simulink model "rcm112_app"  (R2024a)
settings: Solver=FixedStepDiscrete  StartTime=0.0  StopTime=10.0  FixedStep=0.005  RelTol=1e-3  EnableMultiTasking=on
PreLoadFcn:
  | try, model_open; catch, disp('Error occurred while executing model pre-load callback: model_open.m'); disp('Please assure that the MATLAB working directory is set to the model directory before opening.'); end
InitFcn:
  | try, model_open; catch, end
undefined symbols (not defined in the file or in its folder): dataName, enumName, enumValue, raptor_get_safe_string, raptor_xcp_function, RCM
libraries: Raptor_lib x57, simulink x14, simulink_extras x4
(part 2 of 2)

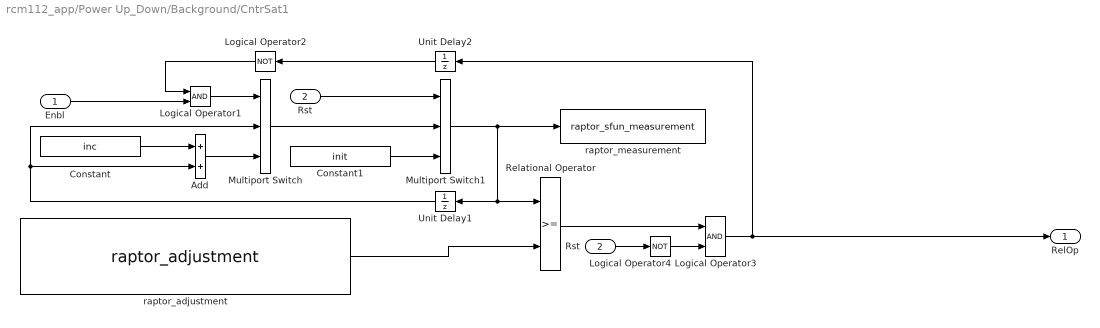
== system rcm112_app/Power Up_Down/Background/CntrSat1 ==
  Enbl : Inport
  Rst : Inport  Port=2
  Add : Sum  InputSameDT=on  OutDataTypeStr=Inherit: Same as first input
  Constant : Constant  Value=inc  OutDataTypeStr=uint32
  Constant1 : Constant  Value=init  OutDataTypeStr=uint32
  Logical Operator1 : Logic  OutDataTypeStr=boolean
  Logical Operator2 : Logic  Operator=NOT  Inputs=1  OutDataTypeStr=boolean
  Logical Operator3 : Logic  OutDataTypeStr=boolean
  Logical Operator4 : Logic  Operator=NOT  Inputs=1  OutDataTypeStr=boolean
  Multiport Switch : MultiPortSwitch  DataPortOrder=Zero-based contiguous  Inputs=2  zeroidx=on  SaturateOnIntegerOverflow=off
  Multiport Switch1 : MultiPortSwitch  DataPortOrder=Zero-based contiguous  Inputs=2  zeroidx=on  SaturateOnIntegerOverflow=off
  Relational Operator : RelationalOperator  OutDataTypeStr=boolean  InputSameDT=off
  "Rst " : InportShadow  Port=2
  Unit Delay1 : UnitDelay  InitialCondition=init  SampleTime=-1  HasFrameUpgradeWarning=on
  Unit Delay2 : UnitDelay  InitialCondition=boolean(0)  SampleTime=-1  HasFrameUpgradeWarning=on
  raptor_adjustment : Raptor_lib/Data Storage/raptor_adjustment  paramName=th_nam  nameSource=Parameter  initValue=timeout / th_gain  dataType=uint32  storage=Calibration  calDispType=Number  calEnum={'Disabled', 'Enabled'}  calGain=th_gain  calOffset=0  calMax=inf  calMin=-inf  calFormat='0.3'  calUnit=th_units  calHelp=th_help  calAccess=4  calFunction=th_group  calDispHeaders=off  calColHeaders={'Col1' 'Col2' 'Col3'}  calRowHeaders={'Row1' 'Row2' 'Row3'}
      settings: SourceProductName=Raptor
  raptor_measurement : S-Function  FunctionName=raptor_sfun_measurement  Parameters=char({dataName,''}), uint8(calDispType), char(enumName), int32(enumValue), double(calGain), double(calOffset), double(calMax), double(calMin), char(calUnit), char(calHelp), char(calFormat), char(calFunction), char(calAccess)  SFunctionDeploymentMode=off  EnableBusSupport=off  mask(Measurement){paramName=[th_nam(1:end-3) 'Tmr'], nameSource=Parameter, calDispType=Number, calEnum={'False', 'True'}, calGain=th_gain, calOffset=0.0, calMax=inf, calMin=-inf, calFormat='0.3', calUnit=th_units, calHelp=['time that gets compared to ' th_nam], calAccess=4, calFunction=th_group, calVisible=on}
      mask prompts: paramName "Name"; nameSource "Name Source"; calDispType "Display as"; calEnum "Enumeration Definition"; calGain "Gain"; calOffset "Offset"; calMax "Max"; calMin "Min"; calFormat "Display Decimal Places"; calUnit "Unit Text"; calHelp "Help Text"; calAccess "Access Level"; calFunction "Function"; calVisible "Visible in Cal"
      mask help: This block is used to display a value in the calibration tool.
      mask init:
      | raptor_sfun_measurement_maskInit;
      settings: MoveFcn=raptor_icon_redraw(gcb);
      mask Help: eval('raptor_help(''raptor_measurement'');')
      mask TypeOptions nameSource: Parameter | Input Wire
      mask Callback nameSource: raptor_sfun_measurement_dlgCb(gcb, 'nameSource');
      mask TypeOptions calDispType: Number | Enumeration | String
      mask Callback calDispType: raptor_sfun_measurement_dlgCb(gcb, 'calDispType');
      mask TypeOptions calAccess: 4 | 3 | 2 | 1
      mask Display: raptor_sfun_measurement_icon;
  RelOp : Outport  VectorParamsAs1DForOutWhenUnconnected=off
  wires:
  "Rst "/1 -> Logical Operator4/1
  Logical Operator4/1 -> Logical Operator3/2
  Relational Operator/1 -> Logical Operator3/1
  Multiport Switch1/1 -> Relational Operator/1, Unit Delay1/1, raptor_measurement/1
  Logical Operator2/1 -> Logical Operator1/1
  Constant1/1 -> Multiport Switch1/3
  Multiport Switch/1 -> Multiport Switch1/2
  Constant/1 -> Add/1
  Unit Delay1/1 -> Multiport Switch/2, Add/2
  Add/1 -> Multiport Switch/3
  Logical Operator1/1 -> Multiport Switch/1
  Enbl/1 -> Logical Operator1/2
  raptor_adjustment/1 -> Relational Operator/2
  Logical Operator3/1 -> RelOp/1, Unit Delay2/1
  Rst/1 -> Multiport Switch1/1
  Unit Delay2/1 -> Logical Operator2/1

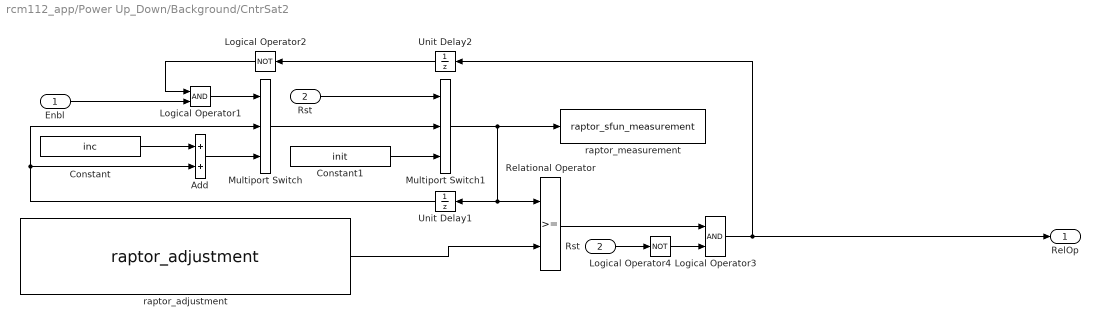
== system rcm112_app/Power Up_Down/Background/CntrSat2 ==
  Enbl : Inport
  Rst : Inport  Port=2
  Add : Sum  InputSameDT=on  OutDataTypeStr=Inherit: Same as first input
  Constant : Constant  Value=inc  OutDataTypeStr=uint32
  Constant1 : Constant  Value=init  OutDataTypeStr=uint32
  Logical Operator1 : Logic  OutDataTypeStr=boolean
  Logical Operator2 : Logic  Operator=NOT  Inputs=1  OutDataTypeStr=boolean
  Logical Operator3 : Logic  OutDataTypeStr=boolean
  Logical Operator4 : Logic  Operator=NOT  Inputs=1  OutDataTypeStr=boolean
  Multiport Switch : MultiPortSwitch  DataPortOrder=Zero-based contiguous  Inputs=2  zeroidx=on  SaturateOnIntegerOverflow=off
  Multiport Switch1 : MultiPortSwitch  DataPortOrder=Zero-based contiguous  Inputs=2  zeroidx=on  SaturateOnIntegerOverflow=off
  Relational Operator : RelationalOperator  OutDataTypeStr=boolean  InputSameDT=off
  "Rst " : InportShadow  Port=2
  Unit Delay1 : UnitDelay  InitialCondition=init  SampleTime=-1  HasFrameUpgradeWarning=on
  Unit Delay2 : UnitDelay  InitialCondition=boolean(0)  SampleTime=-1  HasFrameUpgradeWarning=on
  raptor_adjustment : Raptor_lib/Data Storage/raptor_adjustment  paramName=th_nam  nameSource=Parameter  initValue=timeout / th_gain  dataType=uint32  storage=Calibration  calDispType=Number  calEnum={'Disabled', 'Enabled'}  calGain=th_gain  calOffset=0  calMax=inf  calMin=-inf  calFormat='0.3'  calUnit=th_units  calHelp=th_help  calAccess=4  calFunction=th_group  calDispHeaders=off  calColHeaders={'Col1' 'Col2' 'Col3'}  calRowHeaders={'Row1' 'Row2' 'Row3'}
      settings: SourceProductName=Raptor
  raptor_measurement : S-Function  FunctionName=raptor_sfun_measurement  Parameters=char({dataName,''}), uint8(calDispType), char(enumName), int32(enumValue), double(calGain), double(calOffset), double(calMax), double(calMin), char(calUnit), char(calHelp), char(calFormat), char(calFunction), char(calAccess)  SFunctionDeploymentMode=off  EnableBusSupport=off  mask(Measurement){paramName=[th_nam(1:end-3) 'Tmr'], nameSource=Parameter, calDispType=Number, calEnum={'False', 'True'}, calGain=th_gain, calOffset=0.0, calMax=inf, calMin=-inf, calFormat='0.3', calUnit=th_units, calHelp=['time that gets compared to ' th_nam], calAccess=4, calFunction=th_group, calVisible=on}
      mask prompts: paramName "Name"; nameSource "Name Source"; calDispType "Display as"; calEnum "Enumeration Definition"; calGain "Gain"; calOffset "Offset"; calMax "Max"; calMin "Min"; calFormat "Display Decimal Places"; calUnit "Unit Text"; calHelp "Help Text"; calAccess "Access Level"; calFunction "Function"; calVisible "Visible in Cal"
      mask help: This block is used to display a value in the calibration tool.
      mask init:
      | raptor_sfun_measurement_maskInit;
      settings: MoveFcn=raptor_icon_redraw(gcb);
      mask Help: eval('raptor_help(''raptor_measurement'');')
      mask TypeOptions nameSource: Parameter | Input Wire
      mask Callback nameSource: raptor_sfun_measurement_dlgCb(gcb, 'nameSource');
      mask TypeOptions calDispType: Number | Enumeration | String
      mask Callback calDispType: raptor_sfun_measurement_dlgCb(gcb, 'calDispType');
      mask TypeOptions calAccess: 4 | 3 | 2 | 1
      mask Display: raptor_sfun_measurement_icon;
  RelOp : Outport  VectorParamsAs1DForOutWhenUnconnected=off
  wires:
  "Rst "/1 -> Logical Operator4/1
  Logical Operator4/1 -> Logical Operator3/2
  Relational Operator/1 -> Logical Operator3/1
  Multiport Switch1/1 -> Relational Operator/1, Unit Delay1/1, raptor_measurement/1
  Logical Operator2/1 -> Logical Operator1/1
  Constant1/1 -> Multiport Switch1/3
  Multiport Switch/1 -> Multiport Switch1/2
  Constant/1 -> Add/1
  Unit Delay1/1 -> Multiport Switch/2, Add/2
  Add/1 -> Multiport Switch/3
  Logical Operator1/1 -> Multiport Switch/1
  Enbl/1 -> Logical Operator1/2
  raptor_adjustment/1 -> Relational Operator/2
  Logical Operator3/1 -> RelOp/1, Unit Delay2/1
  Rst/1 -> Multiport Switch1/1
  Unit Delay2/1 -> Logical Operator2/1

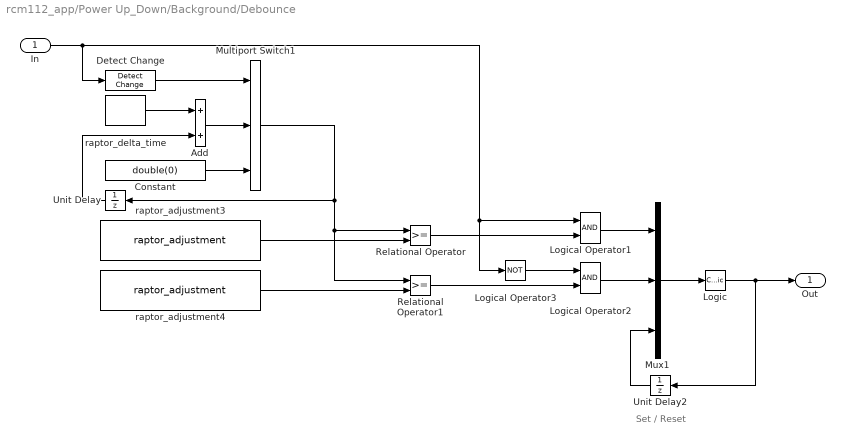
== system rcm112_app/Power Up_Down/Background/Debounce ==
  note: Set / Reset
  In : Inport
  Add : Sum
  Constant : Constant  Value=double(0)
  Detect Change : simulink/Logic and Bit Operations/Detect Change  vinit=0  OutDataTypeStr=boolean
  Logic : CombinatorialLogic  TruthTable=[0;1;0;0;1;1;0;0]
  Logical Operator1 : Logic  AllPortsSameDT=off  OutDataTypeStr=boolean
  Logical Operator2 : Logic  AllPortsSameDT=off  OutDataTypeStr=boolean
  Logical Operator3 : Logic  Operator=NOT  Inputs=1  AllPortsSameDT=off  OutDataTypeStr=boolean
  Multiport Switch1 : MultiPortSwitch  DataPortOrder=Zero-based contiguous  Inputs=2  zeroidx=on  SaturateOnIntegerOverflow=off  InputSameDT=off
  Mux1 : Mux  Inputs=3
  Relational Operator : RelationalOperator  OutDataTypeStr=boolean  InputSameDT=off
  Relational Operator1 : RelationalOperator  OutDataTypeStr=boolean  InputSameDT=off
  Unit Delay : UnitDelay  SampleTime=-1  HasFrameUpgradeWarning=on
  Unit Delay2 : UnitDelay  InitialCondition=1  SampleTime=-1  HasFrameUpgradeWarning=on
  raptor_adjustment3 : Raptor_lib/Data Storage/raptor_adjustment  paramName='KeySwHiTimeThr'  nameSource=Parameter  initValue=0.2  dataType=double  storage=Calibration  calDispType=Number  calEnum={'Active Low', 'Active High'}  calGain=1  calOffset=0  calMax=inf  calMin=-inf  calFormat='-1'  calUnit='sec'  calHelp='State high time threshold'  calAccess=1  calFunction=group  calDispHeaders=off  calColHeaders={'Col1' 'Col2' 'Col3'}  calRowHeaders={'Row1' 'Row2' 'Row3'}
      settings: SourceProductName=Raptor
  raptor_adjustment4 : Raptor_lib/Data Storage/raptor_adjustment  paramName='KeySwLoTimeThr'  nameSource=Parameter  initValue=0.2  dataType=double  storage=Calibration  calDispType=Number  calEnum={'Active Low', 'Active High'}  calGain=1  calOffset=0  calMax=inf  calMin=-inf  calFormat='-1'  calUnit='sec'  calHelp='State low time threshold'  calAccess=1  calFunction=group  calDispHeaders=off  calColHeaders={'Col1' 'Col2' 'Col3'}  calRowHeaders={'Row1' 'Row2' 'Row3'}
      settings: SourceProductName=Raptor
  raptor_delta_time : Raptor_lib/Triggers/raptor_delta_time  unit=seconds
      settings: SourceProductName=Raptor
  Out : Outport  VectorParamsAs1DForOutWhenUnconnected=off
  wires:
  Detect Change/1 -> Multiport Switch1/1
  Logical Operator3/1 -> Logical Operator2/1
  Relational Operator/1 -> Logical Operator1/2
  Logical Operator2/1 -> Mux1/2
  Logical Operator1/1 -> Mux1/1
  Mux1/1 -> Logic/1
  Unit Delay2/1 -> Mux1/3
  In/1 -> Detect Change/1, Logical Operator1/1, Logical Operator3/1
  Multiport Switch1/1 -> Unit Delay/1, Relational Operator/1, Relational Operator1/1
  Add/1 -> Multiport Switch1/2
  Constant/1 -> Multiport Switch1/3
  Relational Operator1/1 -> Logical Operator2/2
  Logic/1 -> Unit Delay2/1, Out/1
  Unit Delay/1 -> Add/2
  raptor_delta_time/1 -> Add/1
  raptor_adjustment4/1 -> Relational Operator1/2
  raptor_adjustment3/1 -> Relational Operator/2

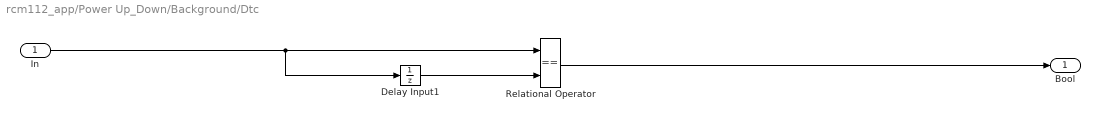
== system rcm112_app/Power Up_Down/Background/Dtc ==
  In : Inport
  Delay Input1 : UnitDelay  Description=Store in Global RAM  DisableCoverage=on  InitialCondition=init  SampleTime=-1  HasFrameUpgradeWarning=on
  Relational Operator : RelationalOperator  Operator===  OutDataTypeStr=boolean
  Bool : Outport  InitialOutput=0  VectorParamsAs1DForOutWhenUnconnected=off
  wires:
  In/1 -> Delay Input1/1, Relational Operator/1
  Delay Input1/1 -> Relational Operator/2
  Relational Operator/1 -> Bool/1

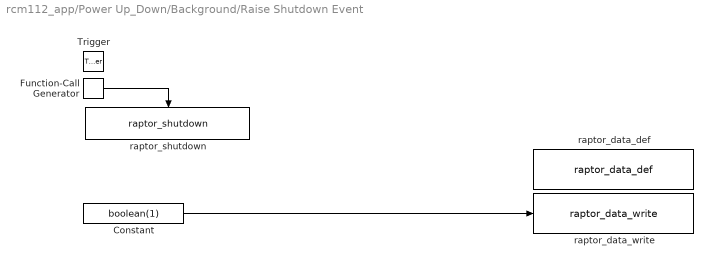
== system rcm112_app/Power Up_Down/Background/Raise Shutdown Event ==
  Trigger : TriggerPort  TriggerType=falling  VariantControl=Variant
  Constant : Constant  Value=boolean(1)
  Function-Call Generator : simulink/Ports & Subsystems/Function-Call Generator  sample_time=-1  numberOfIterations=1  DisallowWideOutput=off
  raptor_data_def : Raptor_lib/Data Storage/raptor_data_def  dataName='FgndTasksStopped'  initValue=0  dataType=boolean  storage=Volatile (RAM)  calVisible=on  calType=Measurement  calDispType=Number  calEnum={'False', 'True'}  calGain=1.0  calOffset=0  calMin=-Inf  calMax=Inf  calFormat='-1'  calUnit='Bool'  calHelp='Boolean indicating foreground tasks stopped'  calAccess=1  calFunction=group  calDispHeaders=off  calColHeaders={'Col1' 'Col2' 'Col3'}  calRowHeaders={'Row1' 'Row2' 'Row3'}
      settings: SourceProductName=Raptor
  raptor_data_write : Raptor_lib/Data Storage/raptor_data_write  dataName='FgndTasksStopped'  dataShape=Scalar  idxSource=Input Port  idxRow=1  idxCol=1
      settings: SourceProductName=Raptor
  raptor_shutdown : Raptor_lib/Triggers/raptor_shutdown  null=0
      settings: SourceProductName=Raptor
  wires:
  Constant/1 -> raptor_data_write/1
  Function-Call Generator/1 -> raptor_shutdown/Trigger

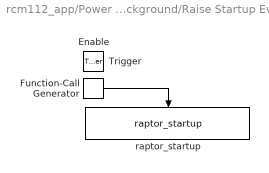
== system rcm112_app/Power Up_Down/Background/Raise Startup Event ==
  Enable : EnablePort
  Trigger : TriggerPort  VariantControl=Variant
  Function-Call Generator : simulink/Ports & Subsystems/Function-Call Generator  sample_time=-1  numberOfIterations=1  DisallowWideOutput=off
  raptor_startup : Raptor_lib/Triggers/raptor_startup  null=0
      settings: SourceProductName=Raptor
  wires:
  Function-Call Generator/1 -> raptor_startup/Trigger

== system rcm112_app/Power Up_Down/Background/Store EEPROM ==
  Enable : EnablePort
  Trigger : TriggerPort  TriggerType=falling  VariantControl=Variant
  Function-Call Generator : simulink/Ports & Subsystems/Function-Call Generator  sample_time=-1  numberOfIterations=1  DisallowWideOutput=off
  raptor_store_nv : Raptor_lib/Data Storage/raptor_store_nv  null=0
      settings: SourceProductName=Raptor
  wires:
  Function-Call Generator/1 -> raptor_store_nv/Trigger
